simulink model "TestBenchModel"  (R2019b)
settings: Solver=VariableStepAuto  StartTime=0.0  StopTime=60  FixedStep=0.0001  RelTol=1e-3  EnableMultiTasking=on
InitFcn:
  | TestBenchData;
StartFcn:
  | TestBenchData;
values from neighbouring files (symbols this model uses):
  C = 0.0056    [TestBenchData.m]
  C1 = C    (= 0.0056)    [TestBenchData.m]
  C2 = C1    (= 0.0056)    [TestBenchData.m]
  C3 = C1    (= 0.0056)    [TestBenchData.m]
  C4 = C1    (= 0.0056)    [TestBenchData.m]
  C5 = C1    (= 0.0056)    [TestBenchData.m]
  C6 = C1    (= 0.0056)    [TestBenchData.m]
  Cfc = 0.35    [TestBenchData.m]
  Fs = 1000    [TestBenchData.m]
  glg = 4    [TestBenchData.m]
  gug = 3    [TestBenchData.m]
  Ic1 = 0.05*10^(-3)    (= 5e-05)    [TestBenchData.m]
  Ic4 = Ic3    (= 0.00012)    [TestBenchData.m]
  Ic_mf = 1.1420e-04    (= 0.0001142)    [TestBenchData.m]
  Ifc_1 = 0.003*10^(-3)    (= 3e-06)    [TestBenchData.m]
  Ifc_2 = 0.003*10^(-3)    (= 3e-06)    [TestBenchData.m]
  Imotor = 0.00068    [TestBenchData.m]
  Iprop = gml^2*I_ML + I_GL + Iprop0    [TestBenchData.m]
  Kc1 = 41.9*10^3    (= 41900)    [TestBenchData.m]
  Kc2 = Kc1    (= 41900)    [TestBenchData.m]
  Kc3 = 31*10^3    (= 31000)    [TestBenchData.m]
  Kc4 = Kc3    (= 31000)    [TestBenchData.m]
  Kc5 = 138*10^3    (= 138000)    [TestBenchData.m]
  Kc6 = Kc5    (= 138000)    [TestBenchData.m]
  Kc_mf = 1.9039e+05    (= 190390)    [TestBenchData.m]
  Kfc = 90    [TestBenchData.m]
  Klg = 44.3*10^3    (= 44300)    [TestBenchData.m]
  Km1 = 5.4*10^3    (= 5400)    [TestBenchData.m]
  Km2 = 20*10^3    (= 20000)    [TestBenchData.m]
  Kug = 43.3*10^3    (= 43300)    [TestBenchData.m]
  lg = C1    (= 0.0056)    [TestBenchData.m]
  M1 = S1    (= 0.0056)    [TestBenchData.m]
  M2 = M1    (= 0.0056)    [TestBenchData.m]
  n = 3221    [TestBenchData.m]
  n_idle = 0    [TestBenchData.m]
  Nmill = 12    [TestBenchData.m]
  P = 1150    [TestBenchData.m]
  prop_blades = 4    [TestBenchData.m]
  S = 0.0056    [TestBenchData.m]
  S1 = S    (= 0.0056)    [TestBenchData.m]
  S2 = S1    (= 0.0056)    [TestBenchData.m]
  S3 = S1    (= 0.0056)    [TestBenchData.m]
  S4 = S1    (= 0.0056)    [TestBenchData.m]
  S5 = S1    (= 0.0056)    [TestBenchData.m]
  T = P/(n/9.55)    (= 3.40965538653)    [TestBenchData.m]
  Tice = 100000    [TestBenchData.m]
  To = 0.2    [TestBenchData.m]
  Todelta = 0.5    [TestBenchData.m]
  ug = C1    (= 0.0056)    [TestBenchData.m]
  W = 131.9469    [TestBenchData.m]
  x4 = 0.06/4    (= 0.015)    [TestBenchData.m]
  x8 = 0.02/4    (= 0.005)    [TestBenchData.m]
  Z = 4    [TestBenchData.m]
  z1 = 17    [TestBenchData.m]
  z2 = 42    [TestBenchData.m]
undefined symbols (not defined in the file or in its folder): C1_22, C1_3, C_crank, C_cyl, Data, Iem, Is1, Is2, Is3, Is4, Is5, K1_11, K1_13, K1_15, K1_21, K1_23, K1_5, K1_7, K1_9, Ks1, Ks2, Ks3, Ks4, Ks5, Ks_mf, RPM, Tu
libraries: fl_lib x201, nesl_utility x92, simulink x22, dspstat3 x1
(part 3 of 3)

== system TestBenchModel/Signals 21 ==
  Ideal Rotational Motion Sensor1 : fl_lib/Mechanical/Mechanical Sensors/Ideal Rotational Motion Sensor  offset=0 rad
  Ideal Torque Sensor1 : fl_lib/Mechanical/Mechanical Sensors/Ideal Torque Sensor
  Mechanical Rotational Reference3 : fl_lib/Mechanical/Rotational Elements/Mechanical Rotational Reference
  PS-Simulink Converter : nesl_utility/PS-Simulink Converter  PhysicalDomain=network_engine_domain  SubClassName=ps_output  LeftPortType=input  RightPortType=output  PseudoPeriodic=off  Frequencies=[]  Unit=N*m  AffineConversion=off
  PS-Simulink Converter1 : nesl_utility/PS-Simulink Converter  PhysicalDomain=network_engine_domain  SubClassName=ps_output  LeftPortType=input  RightPortType=output  PseudoPeriodic=off  Frequencies=[]  Unit=1  AffineConversion=off
  PS-Simulink Converter2 : nesl_utility/PS-Simulink Converter  PhysicalDomain=network_engine_domain  SubClassName=ps_output  LeftPortType=input  RightPortType=output  PseudoPeriodic=off  Frequencies=[]  Unit=1  AffineConversion=off
  in : PMIOPort  Side=Left
  T_out : PMIOPort  Port=2  Side=Right
  tag scope: Angle21=global, AngularSpeed21=global, Torque21=global
  wires:
  PS-Simulink Converter2/1 -> [AngularSpeed21]
  PS-Simulink Converter1/1 -> [Angle21]
  PS-Simulink Converter/1 -> [Torque21]
  connections:
  PS-Simulink Converter1/LConn1 -- Ideal Rotational Motion Sensor1/RConn3
  in/RConn1 -- Ideal Torque Sensor1/LConn1 -- Ideal Rotational Motion Sensor1/LConn1
  PS-Simulink Converter2/LConn1 -- Ideal Rotational Motion Sensor1/RConn2
  Mechanical Rotational Reference3/LConn1 -- Ideal Rotational Motion Sensor1/RConn1
  T_out/RConn1 -- Ideal Torque Sensor1/RConn1
  PS-Simulink Converter/LConn1 -- Ideal Torque Sensor1/RConn2

== system TestBenchModel/Signals 3 ==
  Ideal Rotational Motion Sensor1 : fl_lib/Mechanical/Mechanical Sensors/Ideal Rotational Motion Sensor  offset=0 rad
  Ideal Torque Sensor1 : fl_lib/Mechanical/Mechanical Sensors/Ideal Torque Sensor
  Mechanical Rotational Reference3 : fl_lib/Mechanical/Rotational Elements/Mechanical Rotational Reference
  PS-Simulink Converter : nesl_utility/PS-Simulink Converter  PhysicalDomain=network_engine_domain  SubClassName=ps_output  LeftPortType=input  RightPortType=output  PseudoPeriodic=off  Frequencies=[]  Unit=N*m  AffineConversion=off
  PS-Simulink Converter1 : nesl_utility/PS-Simulink Converter  PhysicalDomain=network_engine_domain  SubClassName=ps_output  LeftPortType=input  RightPortType=output  PseudoPeriodic=off  Frequencies=[]  Unit=1  AffineConversion=off
  PS-Simulink Converter2 : nesl_utility/PS-Simulink Converter  PhysicalDomain=network_engine_domain  SubClassName=ps_output  LeftPortType=input  RightPortType=output  PseudoPeriodic=off  Frequencies=[]  Unit=1  AffineConversion=off
  in : PMIOPort  Side=Left
  T_out : PMIOPort  Port=2  Side=Right
  tag scope: Angle3=global, AngularSpeed3=global, Torque3=global
  wires:
  PS-Simulink Converter/1 -> [Torque3]
  PS-Simulink Converter1/1 -> [Angle3]
  PS-Simulink Converter2/1 -> [AngularSpeed3]
  connections:
  PS-Simulink Converter/LConn1 -- Ideal Torque Sensor1/RConn2
  T_out/RConn1 -- Ideal Torque Sensor1/RConn1
  Mechanical Rotational Reference3/LConn1 -- Ideal Rotational Motion Sensor1/RConn1
  PS-Simulink Converter2/LConn1 -- Ideal Rotational Motion Sensor1/RConn2
  Ideal Rotational Motion Sensor1/LConn1 -- Ideal Torque Sensor1/LConn1 -- in/RConn1
  PS-Simulink Converter1/LConn1 -- Ideal Rotational Motion Sensor1/RConn3

== system TestBenchModel/Signals 4 ==
  Ideal Rotational Motion Sensor1 : fl_lib/Mechanical/Mechanical Sensors/Ideal Rotational Motion Sensor  offset=0 rad
  Ideal Torque Sensor1 : fl_lib/Mechanical/Mechanical Sensors/Ideal Torque Sensor
  Mechanical Rotational Reference3 : fl_lib/Mechanical/Rotational Elements/Mechanical Rotational Reference
  PS-Simulink Converter : nesl_utility/PS-Simulink Converter  PhysicalDomain=network_engine_domain  SubClassName=ps_output  LeftPortType=input  RightPortType=output  PseudoPeriodic=off  Frequencies=[]  Unit=N*m  AffineConversion=off
  PS-Simulink Converter1 : nesl_utility/PS-Simulink Converter  PhysicalDomain=network_engine_domain  SubClassName=ps_output  LeftPortType=input  RightPortType=output  PseudoPeriodic=off  Frequencies=[]  Unit=1  AffineConversion=off
  PS-Simulink Converter2 : nesl_utility/PS-Simulink Converter  PhysicalDomain=network_engine_domain  SubClassName=ps_output  LeftPortType=input  RightPortType=output  PseudoPeriodic=off  Frequencies=[]  Unit=1  AffineConversion=off
  in : PMIOPort  Side=Left
  T_out : PMIOPort  Port=2  Side=Right
  tag scope: Angle4=global, AngularSpeed4=global, Torque4=global
  wires:
  PS-Simulink Converter2/1 -> [AngularSpeed4]
  PS-Simulink Converter1/1 -> [Angle4]
  PS-Simulink Converter/1 -> [Torque4]
  connections:
  PS-Simulink Converter1/LConn1 -- Ideal Rotational Motion Sensor1/RConn3
  in/RConn1 -- Ideal Torque Sensor1/LConn1 -- Ideal Rotational Motion Sensor1/LConn1
  PS-Simulink Converter2/LConn1 -- Ideal Rotational Motion Sensor1/RConn2
  Mechanical Rotational Reference3/LConn1 -- Ideal Rotational Motion Sensor1/RConn1
  T_out/RConn1 -- Ideal Torque Sensor1/RConn1
  PS-Simulink Converter/LConn1 -- Ideal Torque Sensor1/RConn2

== system TestBenchModel/Signals 5 ==
  Ideal Rotational Motion Sensor1 : fl_lib/Mechanical/Mechanical Sensors/Ideal Rotational Motion Sensor  offset=0 rad
  Ideal Torque Sensor1 : fl_lib/Mechanical/Mechanical Sensors/Ideal Torque Sensor
  Mechanical Rotational Reference3 : fl_lib/Mechanical/Rotational Elements/Mechanical Rotational Reference
  PS-Simulink Converter : nesl_utility/PS-Simulink Converter  PhysicalDomain=network_engine_domain  SubClassName=ps_output  LeftPortType=input  RightPortType=output  PseudoPeriodic=off  Frequencies=[]  Unit=N*m  AffineConversion=off
  PS-Simulink Converter1 : nesl_utility/PS-Simulink Converter  PhysicalDomain=network_engine_domain  SubClassName=ps_output  LeftPortType=input  RightPortType=output  PseudoPeriodic=off  Frequencies=[]  Unit=1  AffineConversion=off
  PS-Simulink Converter2 : nesl_utility/PS-Simulink Converter  PhysicalDomain=network_engine_domain  SubClassName=ps_output  LeftPortType=input  RightPortType=output  PseudoPeriodic=off  Frequencies=[]  Unit=1  AffineConversion=off
  in : PMIOPort  Side=Left
  T_out : PMIOPort  Port=2  Side=Right
  tag scope: Angle5=global, AngularSpeed5=global, Torque5=global
  wires:
  PS-Simulink Converter/1 -> [Torque5]
  PS-Simulink Converter1/1 -> [Angle5]
  PS-Simulink Converter2/1 -> [AngularSpeed5]
  connections:
  PS-Simulink Converter/LConn1 -- Ideal Torque Sensor1/RConn2
  T_out/RConn1 -- Ideal Torque Sensor1/RConn1
  Mechanical Rotational Reference3/LConn1 -- Ideal Rotational Motion Sensor1/RConn1
  PS-Simulink Converter2/LConn1 -- Ideal Rotational Motion Sensor1/RConn2
  Ideal Rotational Motion Sensor1/LConn1 -- Ideal Torque Sensor1/LConn1 -- in/RConn1
  PS-Simulink Converter1/LConn1 -- Ideal Rotational Motion Sensor1/RConn3

== system TestBenchModel/Signals 6 ==
  Ideal Rotational Motion Sensor1 : fl_lib/Mechanical/Mechanical Sensors/Ideal Rotational Motion Sensor  offset=0 rad
  Ideal Torque Sensor1 : fl_lib/Mechanical/Mechanical Sensors/Ideal Torque Sensor
  Mechanical Rotational Reference3 : fl_lib/Mechanical/Rotational Elements/Mechanical Rotational Reference
  PS-Simulink Converter : nesl_utility/PS-Simulink Converter  PhysicalDomain=network_engine_domain  SubClassName=ps_output  LeftPortType=input  RightPortType=output  PseudoPeriodic=off  Frequencies=[]  Unit=N*m  AffineConversion=off
  PS-Simulink Converter1 : nesl_utility/PS-Simulink Converter  PhysicalDomain=network_engine_domain  SubClassName=ps_output  LeftPortType=input  RightPortType=output  PseudoPeriodic=off  Frequencies=[]  Unit=1  AffineConversion=off
  PS-Simulink Converter2 : nesl_utility/PS-Simulink Converter  PhysicalDomain=network_engine_domain  SubClassName=ps_output  LeftPortType=input  RightPortType=output  PseudoPeriodic=off  Frequencies=[]  Unit=1  AffineConversion=off
  in : PMIOPort  Side=Left
  T_out : PMIOPort  Port=2  Side=Right
  tag scope: Angle6=global, AngularSpeed6=global, Torque6=global
  wires:
  PS-Simulink Converter2/1 -> [AngularSpeed6]
  PS-Simulink Converter1/1 -> [Angle6]
  PS-Simulink Converter/1 -> [Torque6]
  connections:
  PS-Simulink Converter1/LConn1 -- Ideal Rotational Motion Sensor1/RConn3
  in/RConn1 -- Ideal Torque Sensor1/LConn1 -- Ideal Rotational Motion Sensor1/LConn1
  PS-Simulink Converter2/LConn1 -- Ideal Rotational Motion Sensor1/RConn2
  Mechanical Rotational Reference3/LConn1 -- Ideal Rotational Motion Sensor1/RConn1
  T_out/RConn1 -- Ideal Torque Sensor1/RConn1
  PS-Simulink Converter/LConn1 -- Ideal Torque Sensor1/RConn2

== system TestBenchModel/Signals 7 ==
  Ideal Rotational Motion Sensor1 : fl_lib/Mechanical/Mechanical Sensors/Ideal Rotational Motion Sensor  offset=0 rad
  Ideal Torque Sensor1 : fl_lib/Mechanical/Mechanical Sensors/Ideal Torque Sensor
  Mechanical Rotational Reference3 : fl_lib/Mechanical/Rotational Elements/Mechanical Rotational Reference
  PS-Simulink Converter : nesl_utility/PS-Simulink Converter  PhysicalDomain=network_engine_domain  SubClassName=ps_output  LeftPortType=input  RightPortType=output  PseudoPeriodic=off  Frequencies=[]  Unit=N*m  AffineConversion=off
  PS-Simulink Converter1 : nesl_utility/PS-Simulink Converter  PhysicalDomain=network_engine_domain  SubClassName=ps_output  LeftPortType=input  RightPortType=output  PseudoPeriodic=off  Frequencies=[]  Unit=1  AffineConversion=off
  PS-Simulink Converter2 : nesl_utility/PS-Simulink Converter  PhysicalDomain=network_engine_domain  SubClassName=ps_output  LeftPortType=input  RightPortType=output  PseudoPeriodic=off  Frequencies=[]  Unit=1  AffineConversion=off
  in : PMIOPort  Side=Left
  T_out : PMIOPort  Port=2  Side=Right
  tag scope: Angle7=global, AngularSpeed7=global, Torque7=global
  wires:
  PS-Simulink Converter2/1 -> [AngularSpeed7]
  PS-Simulink Converter1/1 -> [Angle7]
  PS-Simulink Converter/1 -> [Torque7]
  connections:
  PS-Simulink Converter1/LConn1 -- Ideal Rotational Motion Sensor1/RConn3
  in/RConn1 -- Ideal Torque Sensor1/LConn1 -- Ideal Rotational Motion Sensor1/LConn1
  PS-Simulink Converter2/LConn1 -- Ideal Rotational Motion Sensor1/RConn2
  Mechanical Rotational Reference3/LConn1 -- Ideal Rotational Motion Sensor1/RConn1
  T_out/RConn1 -- Ideal Torque Sensor1/RConn1
  PS-Simulink Converter/LConn1 -- Ideal Torque Sensor1/RConn2

== system TestBenchModel/Signals 8 ==
  Ideal Rotational Motion Sensor1 : fl_lib/Mechanical/Mechanical Sensors/Ideal Rotational Motion Sensor  offset=0 rad
  Ideal Torque Sensor1 : fl_lib/Mechanical/Mechanical Sensors/Ideal Torque Sensor
  Mechanical Rotational Reference3 : fl_lib/Mechanical/Rotational Elements/Mechanical Rotational Reference
  PS-Simulink Converter : nesl_utility/PS-Simulink Converter  PhysicalDomain=network_engine_domain  SubClassName=ps_output  LeftPortType=input  RightPortType=output  PseudoPeriodic=off  Frequencies=[]  Unit=N*m  AffineConversion=off
  PS-Simulink Converter1 : nesl_utility/PS-Simulink Converter  PhysicalDomain=network_engine_domain  SubClassName=ps_output  LeftPortType=input  RightPortType=output  PseudoPeriodic=off  Frequencies=[]  Unit=1  AffineConversion=off
  PS-Simulink Converter2 : nesl_utility/PS-Simulink Converter  PhysicalDomain=network_engine_domain  SubClassName=ps_output  LeftPortType=input  RightPortType=output  PseudoPeriodic=off  Frequencies=[]  Unit=1  AffineConversion=off
  in : PMIOPort  Side=Left
  T_out : PMIOPort  Port=2  Side=Right
  tag scope: Angle8=global, AngularSpeed8=global, Torque8=global
  wires:
  PS-Simulink Converter/1 -> [Torque8]
  PS-Simulink Converter1/1 -> [Angle8]
  PS-Simulink Converter2/1 -> [AngularSpeed8]
  connections:
  PS-Simulink Converter/LConn1 -- Ideal Torque Sensor1/RConn2
  T_out/RConn1 -- Ideal Torque Sensor1/RConn1
  Mechanical Rotational Reference3/LConn1 -- Ideal Rotational Motion Sensor1/RConn1
  PS-Simulink Converter2/LConn1 -- Ideal Rotational Motion Sensor1/RConn2
  Ideal Rotational Motion Sensor1/LConn1 -- Ideal Torque Sensor1/LConn1 -- in/RConn1
  PS-Simulink Converter1/LConn1 -- Ideal Rotational Motion Sensor1/RConn3

== system TestBenchModel/Signals 9 ==
  Ideal Rotational Motion Sensor1 : fl_lib/Mechanical/Mechanical Sensors/Ideal Rotational Motion Sensor  offset=0 rad
  Ideal Torque Sensor1 : fl_lib/Mechanical/Mechanical Sensors/Ideal Torque Sensor
  Mechanical Rotational Reference3 : fl_lib/Mechanical/Rotational Elements/Mechanical Rotational Reference
  PS-Simulink Converter : nesl_utility/PS-Simulink Converter  PhysicalDomain=network_engine_domain  SubClassName=ps_output  LeftPortType=input  RightPortType=output  PseudoPeriodic=off  Frequencies=[]  Unit=N*m  AffineConversion=off
  PS-Simulink Converter1 : nesl_utility/PS-Simulink Converter  PhysicalDomain=network_engine_domain  SubClassName=ps_output  LeftPortType=input  RightPortType=output  PseudoPeriodic=off  Frequencies=[]  Unit=1  AffineConversion=off
  PS-Simulink Converter2 : nesl_utility/PS-Simulink Converter  PhysicalDomain=network_engine_domain  SubClassName=ps_output  LeftPortType=input  RightPortType=output  PseudoPeriodic=off  Frequencies=[]  Unit=1  AffineConversion=off
  in : PMIOPort  Side=Left
  T_out : PMIOPort  Port=2  Side=Right
  tag scope: Angle9=global, AngularSpeed9=global, Torque9=global
  wires:
  PS-Simulink Converter2/1 -> [AngularSpeed9]
  PS-Simulink Converter1/1 -> [Angle9]
  PS-Simulink Converter/1 -> [Torque9]
  connections:
  PS-Simulink Converter1/LConn1 -- Ideal Rotational Motion Sensor1/RConn3
  in/RConn1 -- Ideal Torque Sensor1/LConn1 -- Ideal Rotational Motion Sensor1/LConn1
  PS-Simulink Converter2/LConn1 -- Ideal Rotational Motion Sensor1/RConn2
  Mechanical Rotational Reference3/LConn1 -- Ideal Rotational Motion Sensor1/RConn1
  T_out/RConn1 -- Ideal Torque Sensor1/RConn1
  PS-Simulink Converter/LConn1 -- Ideal Torque Sensor1/RConn2

== system TestBenchModel/Signals Motor ==
  Ideal Torque Sensor1 : fl_lib/Mechanical/Mechanical Sensors/Ideal Torque Sensor
  PS-Simulink Converter : nesl_utility/PS-Simulink Converter  PhysicalDomain=network_engine_domain  SubClassName=ps_output  LeftPortType=input  RightPortType=output  PseudoPeriodic=off  Frequencies=[]  Unit=N*m  AffineConversion=off
  in : PMIOPort  Side=Left
  T_out : PMIOPort  Port=2  Side=Right
  tag scope: TorqueMotor=global
  wires:
  PS-Simulink Converter/1 -> [TorqueMotor]
  connections:
  in/RConn1 -- Ideal Torque Sensor1/LConn1
  T_out/RConn1 -- Ideal Torque Sensor1/RConn1
  PS-Simulink Converter/LConn1 -- Ideal Torque Sensor1/RConn2

== system TestBenchModel/Subsystem ==
  T_in : Inport
  K_A2 : Gain  Gain=1/T
  MAXECT1 : simulink/Math Operations/MinMax Running Resettable  Function=max  vinit=0.0
  MAXEGKA1 : simulink/Math Operations/MinMax Running Resettable  Function=max  vinit=0.0
  Mux3 : Mux  Inputs=2
  Mux6 : Mux  Inputs=2
  T_out : Outport
  KA_out : Outport  Port=2
  tag scope: KA_EC_max=global, T_EC_max=global
  wires:
  T_in/1 -> K_A2/1, MAXECT1/1, Mux3/2
  K_A2/1 -> MAXEGKA1/1, Mux6/2  "K_A"
  MAXECT1/1 -> [T_EC_max], Mux3/1
  MAXEGKA1/1 -> Mux6/1, [KA_EC_max]
  Mux3/1 -> T_out/1
  Mux6/1 -> KA_out/1

== system TestBenchModel/Subsystem1 ==
  In3 : Inport
  K_A gear mesh : Gain  Gain=-1/(T*(gug))
  MAXLGKA1 : simulink/Math Operations/MinMax Running Resettable  Function=max  vinit=0.0
  MAXLGT : simulink/Math Operations/MinMax Running Resettable  Function=min  vinit=0.0
  Mux3 : Mux  Inputs=2
  Mux6 : Mux  Inputs=2
  Out1 : Outport
  Out2 : Outport  Port=2
  tag scope: KA_UG_max=global, T_UG_max=global
  wires:
  In3/1 -> MAXLGT/1, Mux3/2, K_A gear mesh/1
  K_A gear mesh/1 -> MAXLGKA1/1, Mux6/2  "K_A"
  MAXLGT/1 -> Mux3/1, [T_UG_max]
  MAXLGKA1/1 -> Mux6/1, [KA_UG_max]
  Mux3/1 -> Out1/1
  Mux6/1 -> Out2/1

== system TestBenchModel/Subsystem2 ==
  In3 : Inport
  K_A gear mesh : Gain  Gain=1/(T*gug*glg)
  MAXLGKA1 : simulink/Math Operations/MinMax Running Resettable  Function=max  vinit=0.0
  MAXLGT : simulink/Math Operations/MinMax Running Resettable  Function=max  vinit=0.0
  Mux3 : Mux  Inputs=2
  Mux6 : Mux  Inputs=2
  Out1 : Outport
  Out2 : Outport  Port=2
  tag scope: KA_LG_max=global, T_LG_max=global
  wires:
  In3/1 -> MAXLGT/1, Mux3/2, K_A gear mesh/1
  K_A gear mesh/1 -> MAXLGKA1/1, Mux6/2  "K_A"
  MAXLGT/1 -> Mux3/1, [T_LG_max]
  MAXLGKA1/1 -> Mux6/1, [KA_LG_max]
  Mux3/1 -> Out1/1
  Mux6/1 -> Out2/1

== system TestBenchModel/Torque sensor ==
  Ideal Torque Sensor1 : fl_lib/Mechanical/Mechanical Sensors/Ideal Torque Sensor
  PS-Simulink Converter : nesl_utility/PS-Simulink Converter  PhysicalDomain=network_engine_domain  SubClassName=ps_output  LeftPortType=input  RightPortType=output  PseudoPeriodic=off  Frequencies=[]  Unit=N*m  AffineConversion=off
  T_in : PMIOPort  Side=Left
  T_out : PMIOPort  Port=2  Side=Right
  signal : Outport
  wires:
  PS-Simulink Converter/1 -> signal/1
  connections:
  PS-Simulink Converter/LConn1 -- Ideal Torque Sensor1/RConn2
  T_in/RConn1 -- Ideal Torque Sensor1/LConn1
  T_out/RConn1 -- Ideal Torque Sensor1/RConn1

== system TestBenchModel/Torque sensor1 ==
  Ideal Torque Sensor1 : fl_lib/Mechanical/Mechanical Sensors/Ideal Torque Sensor
  PS-Simulink Converter : nesl_utility/PS-Simulink Converter  PhysicalDomain=network_engine_domain  SubClassName=ps_output  LeftPortType=input  RightPortType=output  PseudoPeriodic=off  Frequencies=[]  Unit=N*m  AffineConversion=off
  T_in : PMIOPort  Side=Left
  T_out : PMIOPort  Port=2  Side=Right
  signal : Outport
  wires:
  PS-Simulink Converter/1 -> signal/1
  connections:
  PS-Simulink Converter/LConn1 -- Ideal Torque Sensor1/RConn2
  T_in/RConn1 -- Ideal Torque Sensor1/LConn1
  T_out/RConn1 -- Ideal Torque Sensor1/RConn1

== system TestBenchModel/UGrpm ==
  Constant : Constant  Value=9.55
  Ideal Rotational Motion Sensor1 : fl_lib/Mechanical/Mechanical Sensors/Ideal Rotational Motion Sensor  offset=0 rad
  Mechanical Rotational Reference3 : fl_lib/Mechanical/Rotational Elements/Mechanical Rotational Reference
  PS-Simulink Converter1 : nesl_utility/PS-Simulink Converter  PhysicalDomain=network_engine_domain  SubClassName=ps_output  LeftPortType=input  RightPortType=output  PseudoPeriodic=off  Frequencies=[]  Unit=1  AffineConversion=off
  PS-Simulink Converter2 : nesl_utility/PS-Simulink Converter  PhysicalDomain=network_engine_domain  SubClassName=ps_output  LeftPortType=input  RightPortType=output  PseudoPeriodic=off  Frequencies=[]  Unit=1  AffineConversion=off
  Product : Product  RndMeth=Zero
  in : PMIOPort  Side=Left
  vel : Outport
  angle : Outport  Port=2
  wires:
  PS-Simulink Converter1/1 -> angle/1
  PS-Simulink Converter2/1 -> Product/2
  Constant/1 -> Product/1
  Product/1 -> vel/1
  connections:
  Mechanical Rotational Reference3/LConn1 -- Ideal Rotational Motion Sensor1/RConn1
  PS-Simulink Converter2/LConn1 -- Ideal Rotational Motion Sensor1/RConn2
  in/RConn1 -- Ideal Rotational Motion Sensor1/LConn1
  PS-Simulink Converter1/LConn1 -- Ideal Rotational Motion Sensor1/RConn3

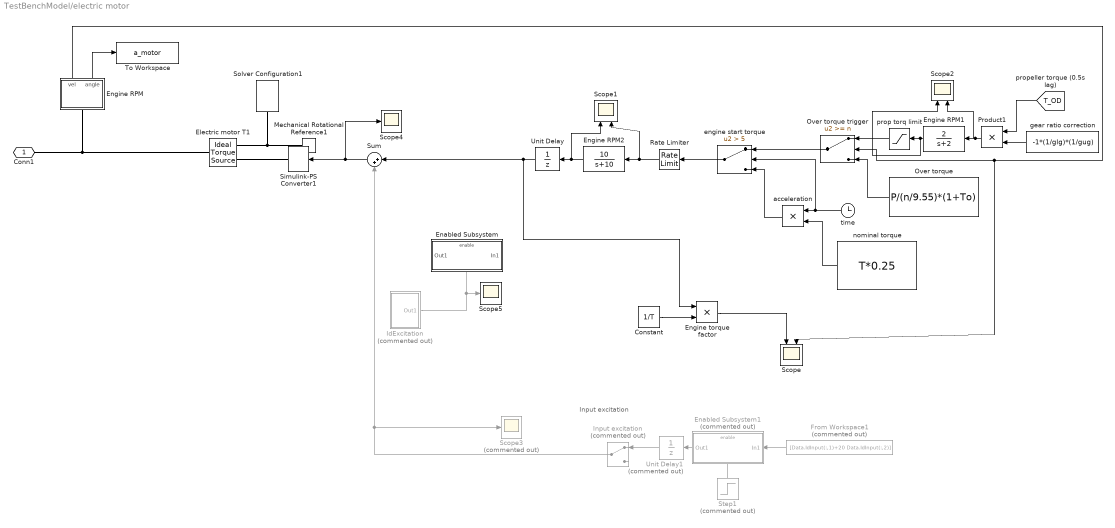
== system TestBenchModel/electric motor ==
  note: Input excitation
  Constant : Constant  Value=1/T
  Electric motor T1 : fl_lib/Mechanical/Mechanical Sources/Ideal Torque Source
  Enabled Subsystem : Subsystem  TreatAsAtomicUnit=on
  Enabled Subsystem1 : Subsystem  Commented=on  TreatAsAtomicUnit=on
  Engine RPM : Subsystem
  Engine RPM1 : TransferFcn  Numerator=[2]  Denominator=[1 2]
  Engine RPM2 : TransferFcn  Numerator=[10]  Denominator=[1 10]
  Engine torque factor : Product  RndMeth=Zero
  From Workspace1 : FromWorkspace  Commented=on  VariableName=[Data.IdInput(:,1)+20 Data.IdInput(:,2)]  SampleTime=0  OutputAfterFinalValue=Setting to zero
  IdExcitation : Subsystem  Commented=on
  Input excitation : ManualSwitch  Commented=on
  Mechanical Rotational Reference1 : fl_lib/Mechanical/Rotational Elements/Mechanical Rotational Reference
  Over torque : Constant  Value=P/(n/9.55)*(1+To)
  Over torque trigger : Switch  Threshold=n
  Product1 : Product  RndMeth=Zero
  Rate Limiter : RateLimiter  RisingSlewLimit=T*Todelta  FallingSlewLimit=-T*(10*Todelta)
  Scope : Scope  NumInputPorts=2
  Scope1 : Scope  NumInputPorts=2
  Scope2 : Scope  NumInputPorts=2
  Scope3 : Scope  Commented=on
  Scope4 : Scope
  Scope5 : Scope
  Simulink-PS Converter1 : nesl_utility/Simulink-PS Converter  PhysicalDomain=network_engine_domain  SubClassName=ps_input  LeftPortType=input  RightPortType=output  PseudoPeriodic=off  Frequencies=[]  NoiseDistribution=none  NoiseParameters=[]  Unit=N*m  AffineConversion=off  FilteringAndDerivatives=zero  SimscapeFilterOrder=1  InputFilterTimeConstant=.001  UdotUserProvided=0
  Solver Configuration1 : nesl_utility/Solver Configuration  PhysicalDomain=network_engine_domain  SubClassName=solver  LeftPortType=input  RightPortType=generic  Tones=[]  Harmonics=[]  SimulateNoise=off  Profile=off  UseLocalSampling=off  EnableSwitchedLinearOptims=on  FrequencyDomain=off  UseCCode=off  RelTol=0.001  AbsTol=1e-06  MinStep=1e-09  ToWorkspace=off  RevertToSquareIcSolve=off  NumHomotopyIterations=100  PhasorMode=off  PhasorModeNumHarmonics=1  DoDC=off  ResidualTolerance=1e-9  UseLocalSolver=on  LocalSolverChoice=NE_BACKWARD_EULER_ADVANCER  LocalSolverSampleTime=.0005  DoFixedCost=on  MaxNonlinIter=20  MaxModeIter=2  LinearAlgebra=Sparse  EquationFormulation=NE_TIME_EF  DelaysMemoryBudget=1024  AutomaticFiltering=on  FilteringTimeConstant=0.0005  PartitionStorageMethod=AS_NEEDED  PartitionMemoryBudget=1024  PartitionMethod=FAST
  Step1 : Step  Commented=on  Time=20  SampleTime=0
  Sum : Sum  Inputs=|++
  To Workspace : ToWorkspace  VariableName=a_motor  SaveFormat=Timeseries  SampleTime=-1
  Unit Delay : UnitDelay  SampleTime=-1  HasFrameUpgradeWarning=on
  Unit Delay1 : UnitDelay  Commented=on  SampleTime=-1  HasFrameUpgradeWarning=on
  acceleration : Product  RndMeth=Zero
  engine start torque : Switch  Criteria=u2 > Threshold  Threshold=5
  gear ratio correction : Constant  Value=-1*(1/glg)*(1/gug)
  nominal torque : Constant  Value=T*0.25
  prop torq limit : Saturate  UpperLimit=T  LowerLimit=0
  time : Clock
  Conn1 : PMIOPort  Side=Left
  wires:
  Constant/1 -> Engine torque factor/2
  time/1 -> acceleration/1, engine start torque/2
  prop torq limit/1 -> Over torque trigger/1
  Engine RPM1/1 -> Scope2/1, prop torq limit/1
  Engine RPM/1(vel) -> Scope/2, Over torque trigger/2
  Engine torque factor/1 -> Scope/1
  Over torque/1 -> Over torque trigger/3
  Product1/1 -> Scope2/2, Engine RPM1/1
  engine start torque/1 -> Rate Limiter/1
  nominal torque/1 -> acceleration/2
  gear ratio correction/1 -> Product1/2
  Rate Limiter/1 -> Scope1/2, Engine RPM2/1
  Engine RPM2/1 -> Scope1/1, Unit Delay/1
  [T_OD] -> Product1/1
  Over torque trigger/1 -> engine start torque/1
  acceleration/1 -> engine start torque/3
  Engine RPM/2(angle) -> To Workspace/1
  Unit Delay/1 -> Sum/1, Engine torque factor/1
  Sum/1 -> Scope4/1, Simulink-PS Converter1/1
  Unit Delay1/1 -> Input excitation/1
  Step1/1 -> Enabled Subsystem1/Enable
  Input excitation/1 -> Scope3/1, Sum/2
  Enabled Subsystem1/1(Out1) -> Unit Delay1/1
  From Workspace1/1 -> Enabled Subsystem1/1(In1)
  IdExcitation/1(Out1) -> Scope5/1, Enabled Subsystem/Enable
  connections:
  Solver Configuration1/RConn1 -- Electric motor T1/RConn2 -- Mechanical Rotational Reference1/LConn1
  Simulink-PS Converter1/RConn1 -- Electric motor T1/RConn1
  Engine RPM/LConn1 -- Electric motor T1/LConn1 -- Conn1/RConn1

== system TestBenchModel/rpm1 ==
  Constant : Constant  Value=9.55
  Ideal Rotational Motion Sensor1 : fl_lib/Mechanical/Mechanical Sensors/Ideal Rotational Motion Sensor  offset=0 rad
  Mechanical Rotational Reference3 : fl_lib/Mechanical/Rotational Elements/Mechanical Rotational Reference
  PS-Simulink Converter1 : nesl_utility/PS-Simulink Converter  PhysicalDomain=network_engine_domain  SubClassName=ps_output  LeftPortType=input  RightPortType=output  PseudoPeriodic=off  Frequencies=[]  Unit=1  AffineConversion=off
  PS-Simulink Converter2 : nesl_utility/PS-Simulink Converter  PhysicalDomain=network_engine_domain  SubClassName=ps_output  LeftPortType=input  RightPortType=output  PseudoPeriodic=off  Frequencies=[]  Unit=1  AffineConversion=off
  Product : Product  RndMeth=Zero
  in : PMIOPort  Side=Left
  vel : Outport
  angle : Outport  Port=2
  wires:
  PS-Simulink Converter1/1 -> angle/1
  PS-Simulink Converter2/1 -> Product/2
  Constant/1 -> Product/1
  Product/1 -> vel/1
  connections:
  Mechanical Rotational Reference3/LConn1 -- Ideal Rotational Motion Sensor1/RConn1
  PS-Simulink Converter2/LConn1 -- Ideal Rotational Motion Sensor1/RConn2
  in/RConn1 -- Ideal Rotational Motion Sensor1/LConn1
  PS-Simulink Converter1/LConn1 -- Ideal Rotational Motion Sensor1/RConn3

== system TestBenchModel/rpm2 ==
  Constant : Constant  Value=9.55
  Ideal Rotational Motion Sensor1 : fl_lib/Mechanical/Mechanical Sensors/Ideal Rotational Motion Sensor  offset=0 rad
  Mechanical Rotational Reference3 : fl_lib/Mechanical/Rotational Elements/Mechanical Rotational Reference
  PS-Simulink Converter1 : nesl_utility/PS-Simulink Converter  PhysicalDomain=network_engine_domain  SubClassName=ps_output  LeftPortType=input  RightPortType=output  PseudoPeriodic=off  Frequencies=[]  Unit=1  AffineConversion=off
  PS-Simulink Converter2 : nesl_utility/PS-Simulink Converter  PhysicalDomain=network_engine_domain  SubClassName=ps_output  LeftPortType=input  RightPortType=output  PseudoPeriodic=off  Frequencies=[]  Unit=1  AffineConversion=off
  Product : Product  RndMeth=Zero
  in : PMIOPort  Side=Left
  vel : Outport
  angle : Outport  Port=2
  wires:
  PS-Simulink Converter1/1 -> angle/1
  PS-Simulink Converter2/1 -> Product/2
  Constant/1 -> Product/1
  Product/1 -> vel/1
  connections:
  Mechanical Rotational Reference3/LConn1 -- Ideal Rotational Motion Sensor1/RConn1
  PS-Simulink Converter2/LConn1 -- Ideal Rotational Motion Sensor1/RConn2
  in/RConn1 -- Ideal Rotational Motion Sensor1/LConn1
  PS-Simulink Converter1/LConn1 -- Ideal Rotational Motion Sensor1/RConn3

== system TestBenchModel/rpm3 ==
  Constant : Constant  Value=9.55
  Ideal Rotational Motion Sensor1 : fl_lib/Mechanical/Mechanical Sensors/Ideal Rotational Motion Sensor  offset=0 rad
  Mechanical Rotational Reference3 : fl_lib/Mechanical/Rotational Elements/Mechanical Rotational Reference
  PS-Simulink Converter1 : nesl_utility/PS-Simulink Converter  PhysicalDomain=network_engine_domain  SubClassName=ps_output  LeftPortType=input  RightPortType=output  PseudoPeriodic=off  Frequencies=[]  Unit=1  AffineConversion=off
  PS-Simulink Converter2 : nesl_utility/PS-Simulink Converter  PhysicalDomain=network_engine_domain  SubClassName=ps_output  LeftPortType=input  RightPortType=output  PseudoPeriodic=off  Frequencies=[]  Unit=1  AffineConversion=off
  Product : Product  RndMeth=Zero
  in : PMIOPort  Side=Left
  vel : Outport
  angle : Outport  Port=2
  wires:
  PS-Simulink Converter1/1 -> angle/1
  PS-Simulink Converter2/1 -> Product/2
  Constant/1 -> Product/1
  Product/1 -> vel/1
  connections:
  Mechanical Rotational Reference3/LConn1 -- Ideal Rotational Motion Sensor1/RConn1
  PS-Simulink Converter2/LConn1 -- Ideal Rotational Motion Sensor1/RConn2
  in/RConn1 -- Ideal Rotational Motion Sensor1/LConn1
  PS-Simulink Converter1/LConn1 -- Ideal Rotational Motion Sensor1/RConn3

== system TestBenchModel/CAT 3512/Flex coupling rpm1 ==
  Constant : Constant  Value=9.55
  Ideal Rotational Motion Sensor1 : fl_lib/Mechanical/Mechanical Sensors/Ideal Rotational Motion Sensor  offset=0 rad
  Mechanical Rotational Reference3 : fl_lib/Mechanical/Rotational Elements/Mechanical Rotational Reference
  PS-Simulink Converter1 : nesl_utility/PS-Simulink Converter  PhysicalDomain=network_engine_domain  SubClassName=ps_output  LeftPortType=input  RightPortType=output  PseudoPeriodic=off  Frequencies=[]  Unit=1  AffineConversion=off
  PS-Simulink Converter2 : nesl_utility/PS-Simulink Converter  PhysicalDomain=network_engine_domain  SubClassName=ps_output  LeftPortType=input  RightPortType=output  PseudoPeriodic=off  Frequencies=[]  Unit=1  AffineConversion=off
  Product : Product  RndMeth=Zero
  in : PMIOPort  Side=Left
  vel : Outport
  angle : Outport  Port=2
  wires:
  PS-Simulink Converter1/1 -> angle/1
  PS-Simulink Converter2/1 -> Product/2
  Constant/1 -> Product/1
  Product/1 -> vel/1
  connections:
  Mechanical Rotational Reference3/LConn1 -- Ideal Rotational Motion Sensor1/RConn1
  PS-Simulink Converter2/LConn1 -- Ideal Rotational Motion Sensor1/RConn2
  in/RConn1 -- Ideal Rotational Motion Sensor1/LConn1
  PS-Simulink Converter1/LConn1 -- Ideal Rotational Motion Sensor1/RConn3

== system TestBenchModel/CAT 3512/Torque sensor ==
  Ideal Torque Sensor1 : fl_lib/Mechanical/Mechanical Sensors/Ideal Torque Sensor
  PS-Simulink Converter : nesl_utility/PS-Simulink Converter  PhysicalDomain=network_engine_domain  SubClassName=ps_output  LeftPortType=input  RightPortType=output  PseudoPeriodic=off  Frequencies=[]  Unit=N*m  AffineConversion=off
  T_in : PMIOPort  Side=Left
  T_out : PMIOPort  Port=2  Side=Right
  signal : Outport
  wires:
  PS-Simulink Converter/1 -> signal/1
  connections:
  PS-Simulink Converter/LConn1 -- Ideal Torque Sensor1/RConn2
  T_in/RConn1 -- Ideal Torque Sensor1/LConn1
  T_out/RConn1 -- Ideal Torque Sensor1/RConn1

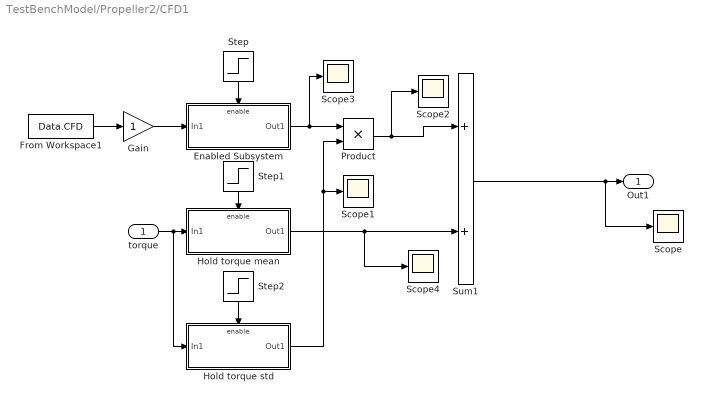
== system TestBenchModel/Propeller2/CFD1 ==
  torque : Inport
  Enabled Subsystem : Subsystem  TreatAsAtomicUnit=on
  From Workspace1 : FromWorkspace  VariableName=Data.CFD  SampleTime=0  OutputAfterFinalValue=Holding final value
  Gain : Gain
  Hold torque mean : Subsystem  TreatAsAtomicUnit=on
  Hold torque std : Subsystem  TreatAsAtomicUnit=on
  Product : Product
  Scope{,1..4} (5 alike) : Scope
  Step : Step  Time=35  SampleTime=0
  Step1 : Step  Time=35  Before=1  After=0  SampleTime=0
  Step2 : Step  Time=35  Before=1  After=0  SampleTime=0
  Sum1 : Sum
  Out1 : Outport
  wires:
  Hold torque std/1(Out1) -> Product/2, Scope1/1
  Product/1 -> Sum1/1, Scope2/1
  Step2/1 -> Hold torque std/Enable
  Sum1/1 -> Out1/1, Scope/1
  Step1/1 -> Hold torque mean/Enable
  torque/1 -> Hold torque mean/1(In1), Hold torque std/1(In1)
  Step/1 -> Enabled Subsystem/Enable
  Enabled Subsystem/1(Out1) -> Scope3/1, Product/1
  From Workspace1/1 -> Gain/1
  Gain/1 -> Enabled Subsystem/1(In1)
  Hold torque mean/1(Out1) -> Scope4/1, Sum1/2

== system TestBenchModel/Propeller2/Enabled Subsystem ==
  In1 : Inport
  Enable : EnablePort
  Out1 : Outport
  wires:
  In1/1 -> Out1/1

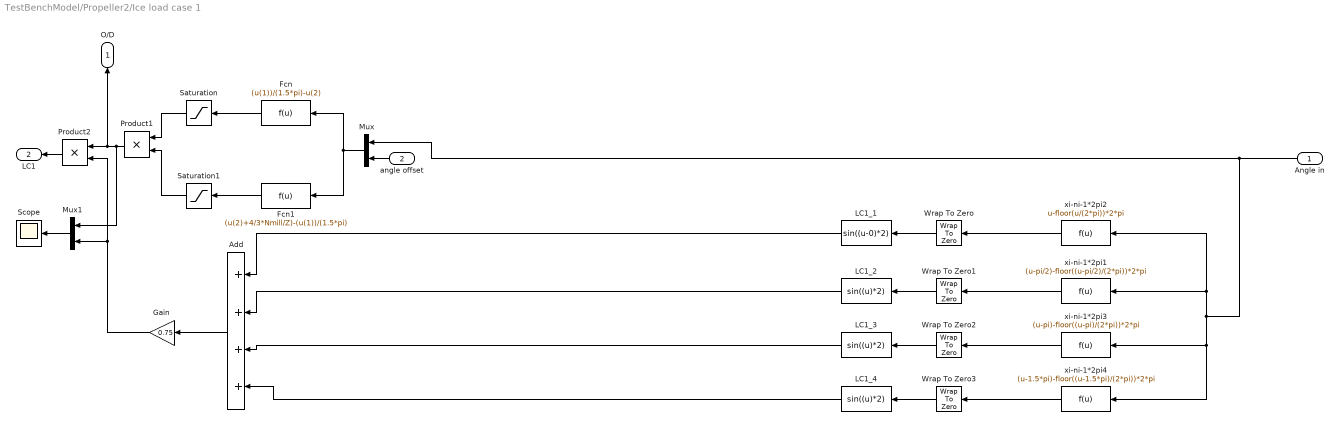
== system TestBenchModel/Propeller2/Ice load case 1 ==
  Angle in : Inport
  angle offset : Inport  Port=2
  Add : Sum  Inputs=++++
  Fcn : Fcn  Expr=(u(1))/(1.5*pi)-u(2)
  Fcn1 : Fcn  Expr=(u(2)+4/3*Nmill/Z)-(u(1))/(1.5*pi)
  Gain : Gain  Gain=0.75
  LC1_1 : Fcn  Expr=sin((u-0)*2)
  LC1_2 : Fcn  Expr=sin((u)*2)
  LC1_3 : Fcn  Expr=sin((u)*2)
  LC1_4 : Fcn  Expr=sin((u)*2)
  Mux : Mux  Inputs=2
  Mux1 : Mux  Inputs=2
  Product1 : Product  RndMeth=Zero
  Product2 : Product  RndMeth=Zero
  Saturation : Saturate  UpperLimit=1  LowerLimit=0
  Saturation1 : Saturate  UpperLimit=1  LowerLimit=0
  Scope : Scope
  Wrap To Zero{,1..3} (4 alike) : simulink/Discontinuities/Wrap To Zero  Threshold=0.5*pi
      settings: SourceProductName=Simulink  SourceProductBaseCode=SL
  xi-ni-1*2pi1 : Fcn  Expr=(u-pi/2)-floor((u-pi/2)/(2*pi))*2*pi
  xi-ni-1*2pi2 : Fcn  Expr=u-floor(u/(2*pi))*2*pi
  xi-ni-1*2pi3 : Fcn  Expr=(u-pi)-floor((u-pi)/(2*pi))*2*pi
  xi-ni-1*2pi4 : Fcn  Expr=(u-1.5*pi)-floor((u-1.5*pi)/(2*pi))*2*pi
  O/D : Outport
  LC1 : Outport  Port=2
  wires:
  Fcn/1 -> Saturation/1
  Saturation/1 -> Product1/1
  Fcn1/1 -> Saturation1/1
  Saturation1/1 -> Product1/2
  Product1/1 -> Product2/1, O/D/1, Mux1/1
  Add/1 -> Gain/1
  Mux/1 -> Fcn/1, Fcn1/1
  Angle in/1 -> Mux/1, xi-ni-1*2pi2/1, xi-ni-1*2pi1/1, xi-ni-1*2pi3/1, xi-ni-1*2pi4/1
  Product2/1 -> LC1/1
  angle offset/1 -> Mux/2
  xi-ni-1*2pi2/1 -> Wrap To Zero/1
  Wrap To Zero/1 -> LC1_1/1
  Wrap To Zero1/1 -> LC1_2/1
  xi-ni-1*2pi1/1 -> Wrap To Zero1/1
  Wrap To Zero2/1 -> LC1_3/1
  xi-ni-1*2pi3/1 -> Wrap To Zero2/1
  LC1_1/1 -> Add/1
  LC1_2/1 -> Add/2
  LC1_3/1 -> Add/3
  Wrap To Zero3/1 -> LC1_4/1
  xi-ni-1*2pi4/1 -> Wrap To Zero3/1
  LC1_4/1 -> Add/4
  Gain/1 -> Product2/2, Mux1/2
  Mux1/1 -> Scope/1

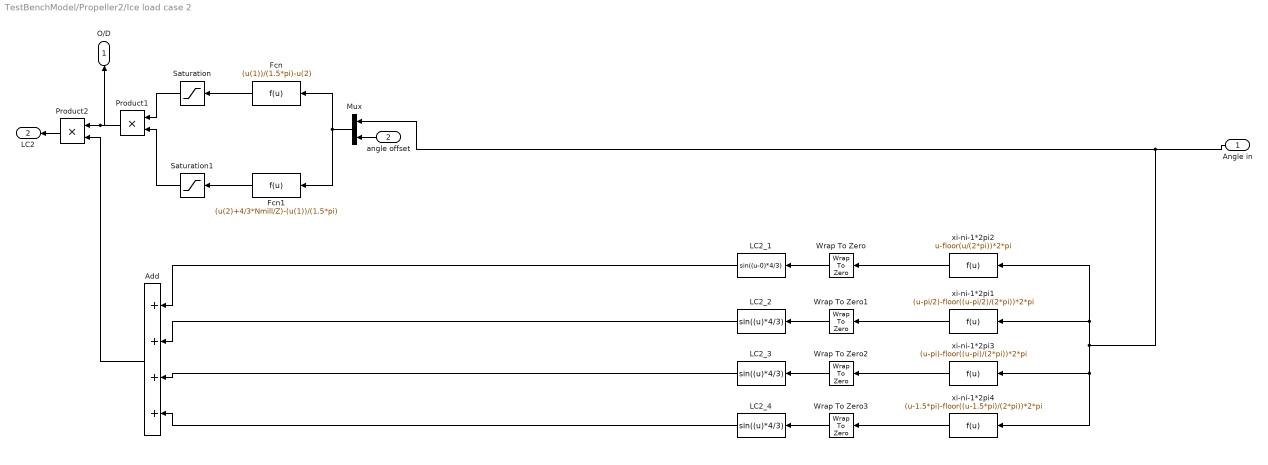
== system TestBenchModel/Propeller2/Ice load case 2 ==
  Angle in : Inport
  angle offset : Inport  Port=2
  Add : Sum  Inputs=++++
  Fcn : Fcn  Expr=(u(1))/(1.5*pi)-u(2)
  Fcn1 : Fcn  Expr=(u(2)+4/3*Nmill/Z)-(u(1))/(1.5*pi)
  LC2_1 : Fcn  Expr=sin((u-0)*4/3)
  LC2_2 : Fcn  Expr=sin((u)*4/3)
  LC2_3 : Fcn  Expr=sin((u)*4/3)
  LC2_4 : Fcn  Expr=sin((u)*4/3)
  Mux : Mux  Inputs=2
  Product1 : Product  RndMeth=Zero
  Product2 : Product  RndMeth=Zero
  Saturation : Saturate  UpperLimit=1  LowerLimit=0
  Saturation1 : Saturate  UpperLimit=1  LowerLimit=0
  Wrap To Zero{,1..3} (4 alike) : simulink/Discontinuities/Wrap To Zero  Threshold=3/4*pi
      settings: SourceProductName=Simulink  SourceProductBaseCode=SL
  xi-ni-1*2pi1 : Fcn  Expr=(u-pi/2)-floor((u-pi/2)/(2*pi))*2*pi
  xi-ni-1*2pi2 : Fcn  Expr=u-floor(u/(2*pi))*2*pi
  xi-ni-1*2pi3 : Fcn  Expr=(u-pi)-floor((u-pi)/(2*pi))*2*pi
  xi-ni-1*2pi4 : Fcn  Expr=(u-1.5*pi)-floor((u-1.5*pi)/(2*pi))*2*pi
  O/D : Outport
  LC2 : Outport  Port=2
  wires:
  Fcn/1 -> Saturation/1
  Saturation/1 -> Product1/1
  Fcn1/1 -> Saturation1/1
  Saturation1/1 -> Product1/2
  Product1/1 -> Product2/1, O/D/1
  Mux/1 -> Fcn/1, Fcn1/1
  Angle in/1 -> Mux/1, xi-ni-1*2pi2/1, xi-ni-1*2pi1/1, xi-ni-1*2pi3/1, xi-ni-1*2pi4/1
  Product2/1 -> LC2/1
  angle offset/1 -> Mux/2
  xi-ni-1*2pi2/1 -> Wrap To Zero/1
  Wrap To Zero/1 -> LC2_1/1
  Wrap To Zero1/1 -> LC2_2/1
  xi-ni-1*2pi1/1 -> Wrap To Zero1/1
  Wrap To Zero2/1 -> LC2_3/1
  xi-ni-1*2pi3/1 -> Wrap To Zero2/1
  LC2_1/1 -> Add/1
  LC2_2/1 -> Add/2
  LC2_3/1 -> Add/3
  Wrap To Zero3/1 -> LC2_4/1
  xi-ni-1*2pi4/1 -> Wrap To Zero3/1
  LC2_4/1 -> Add/4
  Add/1 -> Product2/2

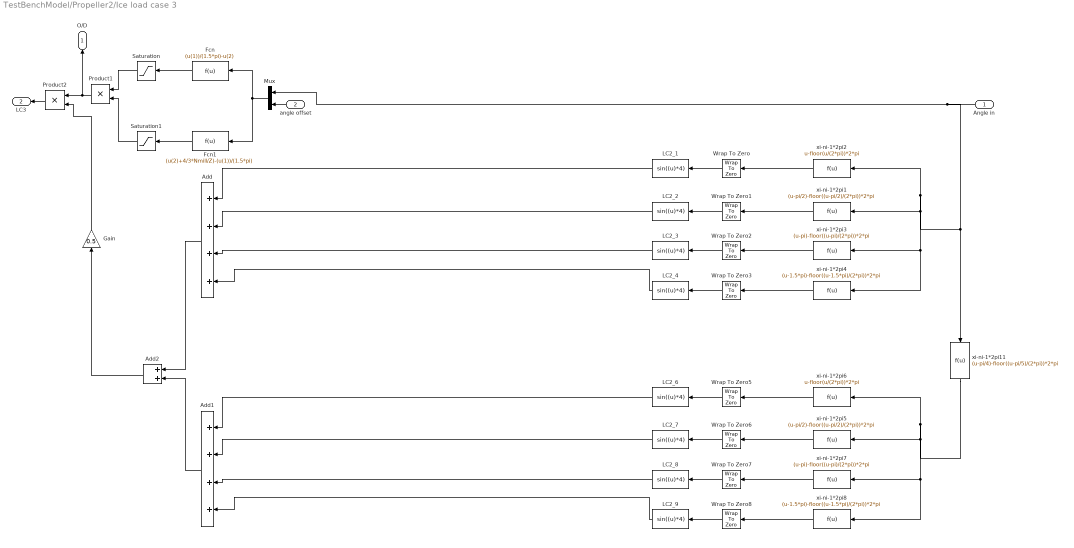
== system TestBenchModel/Propeller2/Ice load case 3 ==
  Angle in : Inport
  angle offset : Inport  Port=2
  Add : Sum  Inputs=++++
  Add1 : Sum  Inputs=++++
  Add2 : Sum
  Fcn : Fcn  Expr=(u(1))/(1.5*pi)-u(2)
  Fcn1 : Fcn  Expr=(u(2)+4/3*Nmill/Z)-(u(1))/(1.5*pi)
  Gain : Gain  Gain=0.5
  LC2_{1..4,6..9} (8 alike) : Fcn  Expr=sin((u)*4)
  Mux : Mux  Inputs=2
  Product1 : Product  RndMeth=Zero
  Product2 : Product  RndMeth=Zero
  Saturation : Saturate  UpperLimit=1  LowerLimit=0
  Saturation1 : Saturate  UpperLimit=1  LowerLimit=0
  Wrap To Zero{,1..3,5..8} (8 alike) : simulink/Discontinuities/Wrap To Zero  Threshold=1/4*pi
      settings: SourceProductName=Simulink  SourceProductBaseCode=SL
  xi-ni-1*2pi1 : Fcn  Expr=(u-pi/2)-floor((u-pi/2)/(2*pi))*2*pi
  xi-ni-1*2pi11 : Fcn  Expr=(u-pi/4)-floor((u-pi/5)/(2*pi))*2*pi
  xi-ni-1*2pi2 : Fcn  Expr=u-floor(u/(2*pi))*2*pi
  xi-ni-1*2pi3 : Fcn  Expr=(u-pi)-floor((u-pi)/(2*pi))*2*pi
  xi-ni-1*2pi4 : Fcn  Expr=(u-1.5*pi)-floor((u-1.5*pi)/(2*pi))*2*pi
  xi-ni-1*2pi5 : Fcn  Expr=(u-pi/2)-floor((u-pi/2)/(2*pi))*2*pi
  xi-ni-1*2pi6 : Fcn  Expr=u-floor(u/(2*pi))*2*pi
  xi-ni-1*2pi7 : Fcn  Expr=(u-pi)-floor((u-pi)/(2*pi))*2*pi
  xi-ni-1*2pi8 : Fcn  Expr=(u-1.5*pi)-floor((u-1.5*pi)/(2*pi))*2*pi
  O/D : Outport
  LC3 : Outport  Port=2
  wires:
  Fcn/1 -> Saturation/1
  Saturation/1 -> Product1/1
  Fcn1/1 -> Saturation1/1
  Saturation1/1 -> Product1/2
  Product1/1 -> Product2/1, O/D/1
  Mux/1 -> Fcn/1, Fcn1/1
  Angle in/1 -> Mux/1, xi-ni-1*2pi1/1, xi-ni-1*2pi3/1, xi-ni-1*2pi4/1, xi-ni-1*2pi2/1, xi-ni-1*2pi11/1
  Product2/1 -> LC3/1
  angle offset/1 -> Mux/2
  xi-ni-1*2pi2/1 -> Wrap To Zero/1
  xi-ni-1*2pi1/1 -> Wrap To Zero1/1
  xi-ni-1*2pi3/1 -> Wrap To Zero2/1
  LC2_1/1 -> Add/1
  LC2_2/1 -> Add/2
  LC2_3/1 -> Add/3
  xi-ni-1*2pi4/1 -> Wrap To Zero3/1
  LC2_4/1 -> Add/4
  Wrap To Zero3/1 -> LC2_4/1
  Wrap To Zero2/1 -> LC2_3/1
  Wrap To Zero1/1 -> LC2_2/1
  Wrap To Zero/1 -> LC2_1/1
  xi-ni-1*2pi6/1 -> Wrap To Zero5/1
  xi-ni-1*2pi5/1 -> Wrap To Zero6/1
  xi-ni-1*2pi7/1 -> Wrap To Zero7/1
  LC2_6/1 -> Add1/1
  LC2_7/1 -> Add1/2
  LC2_8/1 -> Add1/3
  xi-ni-1*2pi8/1 -> Wrap To Zero8/1
  LC2_9/1 -> Add1/4
  Wrap To Zero8/1 -> LC2_9/1
  Wrap To Zero7/1 -> LC2_8/1
  Wrap To Zero6/1 -> LC2_7/1
  Wrap To Zero5/1 -> LC2_6/1
  xi-ni-1*2pi11/1 -> xi-ni-1*2pi8/1, xi-ni-1*2pi7/1, xi-ni-1*2pi5/1, xi-ni-1*2pi6/1
  Add1/1 -> Add2/2
  Add/1 -> Add2/1
  Add2/1 -> Gain/1
  Gain/1 -> Product2/2

== system TestBenchModel/Propeller2/Over torque trigger ==
  O/D in : Inport
  Transport Delay3 : TransportDelay  DelayTime=0.0
  tag scope: T_OD=global
  wires:
  Transport Delay3/1 -> [T_OD]
  O/D in/1 -> Transport Delay3/1

== system TestBenchModel/Propeller2/Propeller excitation order 4 ==
  Angle in : Inport
  Gain : Gain  Gain=x4
  LC1_1 : Fcn  Expr=sin((u)*prop_blades)
  Scope : Scope
  Prop 1 : Outport
  wires:
  Angle in/1 -> LC1_1/1
  Gain/1 -> Scope/1, Prop 1/1
  LC1_1/1 -> Gain/1

== system TestBenchModel/Propeller2/Propeller excitation order 8 ==
  Angle in : Inport
  Gain : Gain  Gain=x8
  LC1_1 : Fcn  Expr=sin((u)*8)
  Scope : Scope
  Prop 2 : Outport
  wires:
  Gain/1 -> Scope/1, Prop 2/1
  Angle in/1 -> LC1_1/1
  LC1_1/1 -> Gain/1

== system TestBenchModel/Propeller2/Signals 22  ==
  Ideal Rotational Motion Sensor1 : fl_lib/Mechanical/Mechanical Sensors/Ideal Rotational Motion Sensor  offset=0 rad
  Ideal Torque Sensor1 : fl_lib/Mechanical/Mechanical Sensors/Ideal Torque Sensor
  Mechanical Rotational Reference3 : fl_lib/Mechanical/Rotational Elements/Mechanical Rotational Reference
  PS-Simulink Converter : nesl_utility/PS-Simulink Converter  PhysicalDomain=network_engine_domain  SubClassName=ps_output  LeftPortType=input  RightPortType=output  PseudoPeriodic=off  Frequencies=[]  Unit=N*m  AffineConversion=off
  PS-Simulink Converter1 : nesl_utility/PS-Simulink Converter  PhysicalDomain=network_engine_domain  SubClassName=ps_output  LeftPortType=input  RightPortType=output  PseudoPeriodic=off  Frequencies=[]  Unit=1  AffineConversion=off
  PS-Simulink Converter2 : nesl_utility/PS-Simulink Converter  PhysicalDomain=network_engine_domain  SubClassName=ps_output  LeftPortType=input  RightPortType=output  PseudoPeriodic=off  Frequencies=[]  Unit=1  AffineConversion=off
  in : PMIOPort  Side=Left
  T_out : PMIOPort  Port=2  Side=Right
  tag scope: Angle22=global, AngularSpeed22=global, TorquePropeller=global
  wires:
  PS-Simulink Converter2/1 -> [AngularSpeed22]
  PS-Simulink Converter1/1 -> [Angle22]
  PS-Simulink Converter/1 -> [TorquePropeller]
  connections:
  PS-Simulink Converter1/LConn1 -- Ideal Rotational Motion Sensor1/RConn3
  in/RConn1 -- Ideal Torque Sensor1/LConn1 -- Ideal Rotational Motion Sensor1/LConn1
  PS-Simulink Converter2/LConn1 -- Ideal Rotational Motion Sensor1/RConn2
  Mechanical Rotational Reference3/LConn1 -- Ideal Rotational Motion Sensor1/RConn1
  T_out/RConn1 -- Ideal Torque Sensor1/RConn1
  PS-Simulink Converter/LConn1 -- Ideal Torque Sensor1/RConn2

== system TestBenchModel/electric motor/Enabled Subsystem ==
  In1 : Inport
  Enable : EnablePort
  Out1 : Outport
  wires:
  In1/1 -> Out1/1

== system TestBenchModel/electric motor/Enabled Subsystem1 ==
  In1 : Inport
  Enable : EnablePort
  Out1 : Outport
  wires:
  In1/1 -> Out1/1

== system TestBenchModel/electric motor/Engine RPM ==
  Constant : Constant  Value=9.55
  Ideal Rotational Motion Sensor1 : fl_lib/Mechanical/Mechanical Sensors/Ideal Rotational Motion Sensor  offset=0 rad
  Mechanical Rotational Reference3 : fl_lib/Mechanical/Rotational Elements/Mechanical Rotational Reference
  PS-Simulink Converter1 : nesl_utility/PS-Simulink Converter  PhysicalDomain=network_engine_domain  SubClassName=ps_output  LeftPortType=input  RightPortType=output  PseudoPeriodic=off  Frequencies=[]  Unit=1  AffineConversion=off
  PS-Simulink Converter2 : nesl_utility/PS-Simulink Converter  PhysicalDomain=network_engine_domain  SubClassName=ps_output  LeftPortType=input  RightPortType=output  PseudoPeriodic=off  Frequencies=[]  Unit=1  AffineConversion=off
  Product : Product  RndMeth=Zero
  in : PMIOPort  Side=Left
  vel : Outport
  angle : Outport  Port=2
  wires:
  PS-Simulink Converter1/1 -> angle/1
  PS-Simulink Converter2/1 -> Product/2
  Constant/1 -> Product/1
  Product/1 -> vel/1
  connections:
  Mechanical Rotational Reference3/LConn1 -- Ideal Rotational Motion Sensor1/RConn1
  PS-Simulink Converter2/LConn1 -- Ideal Rotational Motion Sensor1/RConn2
  in/RConn1 -- Ideal Rotational Motion Sensor1/LConn1
  PS-Simulink Converter1/LConn1 -- Ideal Rotational Motion Sensor1/RConn3

== system TestBenchModel/electric motor/IdExcitation ==
  Step : Step  Time=20  Before=1  After=0  SampleTime=0
  Step2 : Step  Time=20+Data.IdTmax  SampleTime=0
  Sum : Sum  Inputs=|++
  Out1 : Outport
  wires:
  Step2/1 -> Sum/2
  Step/1 -> Sum/1
  Sum/1 -> Out1/1

== system TestBenchModel/Propeller2/CFD1/Enabled Subsystem ==
  In1 : Inport
  Enable : EnablePort
  Out1 : Outport
  wires:
  In1/1 -> Out1/1

== system TestBenchModel/Propeller2/CFD1/Hold torque mean ==
  In1 : Inport
  Enable : EnablePort
  Out1 : Outport
  wires:
  In1/1 -> Out1/1

== system TestBenchModel/Propeller2/CFD1/Hold torque std ==
  In1 : Inport
  Enable : EnablePort
  Moving Standard Deviation : dspstat3/Moving Standard Deviation  Method=Sliding window  ForgettingFactorPort=off  SpecifyWindowLength=on  WindowLength=1000  ForgettingFactor=0.9  SimulateUsing=Code generation
      settings: SourceProductName=DSP System Toolbox  SourceProductBaseCode=DS
  Scope : Scope
  Out1 : Outport
  wires:
  Moving Standard Deviation/1 -> Out1/1, Scope/1
  In1/1 -> Moving Standard Deviation/1
